simulink model "case_24_mode_231"  (R2025b)
settings: Solver=VariableStepAuto  StartTime=0.0  StopTime=20  RelTol=1e-3
settings Model: Creator=sanborkl  LastModifiedBy=admin

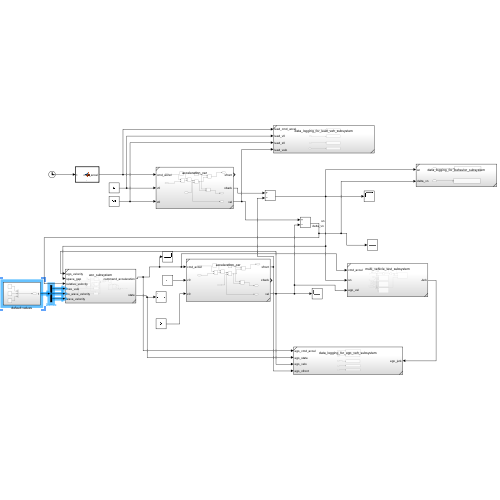
[thumbnail: Simulink's stored preview of the top-level diagram]
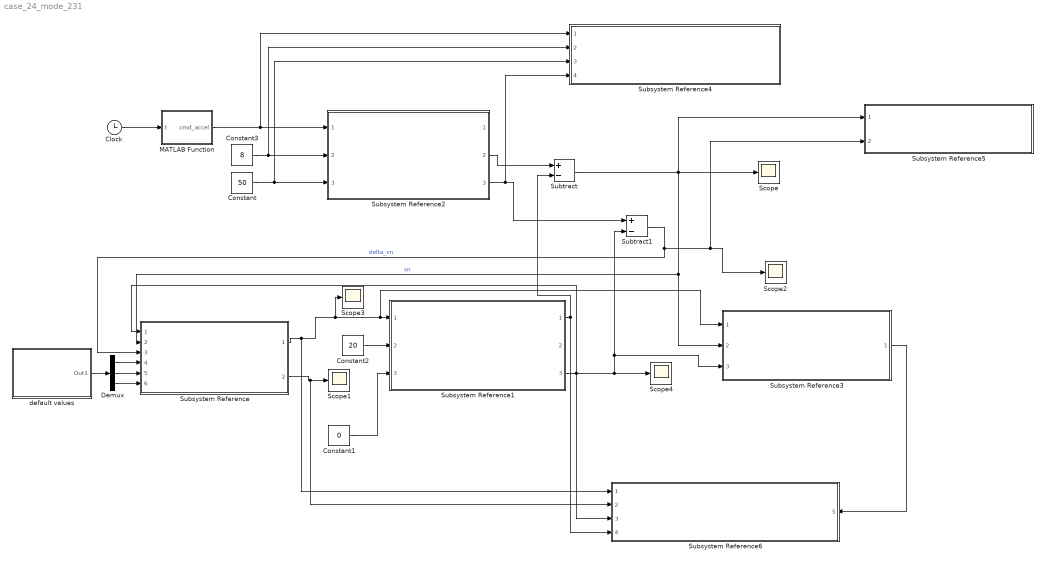
== system case_24_mode_231 ==
  Clock : Clock
  Constant : Constant  Value=50
  Constant1 : Constant  Value=0
  Constant2 : Constant  Value=20
  Constant3 : Constant  Value=8
  Demux : Demux  Outputs=3
  MATLAB Function : MATLAB Function  TreatAsAtomicUnit=on
  Scope{,1..4} (5 alike) : Scope
      Scope settings: ActiveDisplayYMinimum=-1  ActiveDisplayYMaximum=1
      Scope1 settings: ActiveDisplayYMinimum=-0.37499999999999989  ActiveDisplayYMaximum=3.375  DataLoggingVariableName=ScopeData2
      Scope2 settings: ActiveDisplayYMinimum=-10.624999999999998  ActiveDisplayYMaximum=95.625  DataLoggingVariableName=ScopeData3
      Scope3 settings: ActiveDisplayYMinimum=-0.4809516982343458  ActiveDisplayYMaximum=1.9609302395128785  DataLoggingVariableName=ScopeData4
      Scope4 settings: ActiveDisplayYMinimum=18.125  ActiveDisplayYMaximum=36.875
  Subsystem Reference : Subsystem  ReferencedSubsystem=acc_subsystem
  Subsystem Reference1 : Subsystem  ReferencedSubsystem=acceleration_car
  Subsystem Reference2 : Subsystem  ReferencedSubsystem=acceleration_car
  Subsystem Reference3 : Subsystem  ReferencedSubsystem=multi_vehicle_test_subsystem
  Subsystem Reference4 : Subsystem  ReferencedSubsystem=data_logging_for_lead_veh_subsystem
  Subsystem Reference5 : Subsystem  ReferencedSubsystem=data_logging_for_behavior_subsystem
  Subsystem Reference6 : Subsystem  ReferencedSubsystem=data_logging_for_ego_veh_subsystem
      settings: PortSchema="{\"entries\":[{\"content\":{\"sides\":[{\"content\":{\"connectorIds\":[\"In1\",\"In2\",\"In3\",\"In4\"]},\"type\":\"ConnectorPlacement.EquallySpacedRectSide\",\"uuid\":\"1bb3a8cf-f981-4f8a-aff9-03896ccf7d7c\"},{\"content\":{\"connectorIds\":[\"In5\"],\"side\":\"RIGHT\"},\"type\":\"ConnectorPlacement.EquallySpacedRectSide\",\"uuid\":\"3f6ac5cb-96be-44a3-8993-3635a91bd658\"},{\"content\":{\"side\":\"TOP\"},\"type\":\"ConnectorPlacement.EquallySpacedRectSide\",\"uuid\":\"c641fc7f-a424-4033-b273-2526f6b205c0\"}]},\"type\":\"ConnectorPlacement.EquallySpacedConnector\",\"uuid\":\"2a4be48e-084e-4aa6-b74f-8fe234fedc1a\"}],\"packageUris\":[\"http://schema.mathworks.com/mf0/Connector/R2020b\"],\"version\":\"1.0\"}"
  Subtract : Sum  Inputs=+-
  Subtract1 : Sum  Inputs=+-
  default values : Subsystem
  wires:
  Subsystem Reference/1 -> Subsystem Reference6/1, Scope3/1, Subsystem Reference3/1, Subsystem Reference1/1
  Subsystem Reference1/1 -> Subtract/2, Subsystem Reference6/4
  Subsystem Reference/2 -> Subsystem Reference6/2, Scope1/1
  MATLAB Function/1(cmd_accel) -> Subsystem Reference4/1, Subsystem Reference2/1
  Clock/1 -> MATLAB Function/1(t)
  Constant1/1 -> Subsystem Reference1/3
  Subsystem Reference3/1 -> Subsystem Reference6/5
  Subsystem Reference2/2 -> Subtract/1
  Subsystem Reference2/3 -> Subsystem Reference4/4, Subtract1/1
  Constant2/1 -> Subsystem Reference1/2
  Subsystem Reference1/3 -> Subtract1/2, Subsystem Reference3/3, Scope4/1, Subsystem Reference6/3, Subsystem Reference/1
  Constant/1 -> Subsystem Reference4/3, Subsystem Reference2/3
  Subtract1/1 -> Subsystem Reference5/2, Scope2/1, Subsystem Reference/3  "delta_vn"
  Constant3/1 -> Subsystem Reference4/2, Subsystem Reference2/2
  Subtract/1 -> Subsystem Reference5/1, Subsystem Reference3/2, Subsystem Reference/2, Scope/1  "sn"
  Demux/3 -> Subsystem Reference/6
  Demux/2 -> Subsystem Reference/5
  default values/1(Out1) -> Demux/1
  Demux/1 -> Subsystem Reference/4

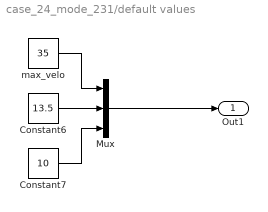
== system case_24_mode_231/default values ==
  Constant6 : Constant  Value=13.5
  Constant7 : Constant  Value=10
  Mux : Mux  Inputs=3
  max_velo : Constant  Value=35
  Out1 : Outport
  wires:
  Constant7/1 -> Mux/3
  Constant6/1 -> Mux/2
  max_velo/1 -> Mux/1
  Mux/1 -> Out1/1

== matlab function case_24_mode_231/MATLAB Function ==
  data: t input; cmd_accel output
function cmd_accel = fcn(t)

if t < 4
    cmd_accel = 0;
elseif t >= 4 && t < 10
    cmd_accel = 0.75;
elseif t >= 10 && t < 15
    cmd_accel = -0.5;
else
    cmd_accel = 0;
end
